simulink library "nonlinearPlnt_cl"  (R2018a)
settings: Solver=VariableStepAuto  StartTime=0.0  StopTime=10.0  RelTol=1e-3
libraries: nonlinearPlnt_ul x1
settings Model: Creator=mcobb  LastModifiedBy=mcobb

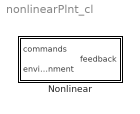
== system nonlinearPlnt_cl ==
  Nonlinear : Subsystem  VariantControl=VSS_NONLINEAR_PLNT

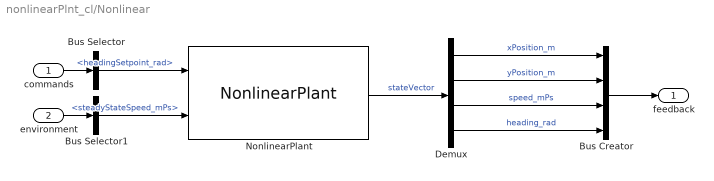
== system nonlinearPlnt_cl/Nonlinear ==
  commands : Inport
  environment : Inport  Port=2
  Bus Creator : BusCreator  Inputs=4
  Bus Selector : BusSelector  OutputSignals=headingSetpoint_rad
  Bus Selector1 : BusSelector  OutputSignals=steadyStateSpeed_mPs
  Demux : Demux
  NonlinearPlant : nonlinearPlnt_ul/NonlinearPlant
  feedback : Outport
  wires:
  Bus Selector1/1 -> NonlinearPlant/2  "<steadyStateSpeed_mPs>"
  Bus Selector/1 -> NonlinearPlant/1  "<headingSetpoint_rad>"
  commands/1 -> Bus Selector/1
  environment/1 -> Bus Selector1/1
  Bus Creator/1 -> feedback/1
  NonlinearPlant/1 -> Demux/1  "stateVector"
  Demux/1 -> Bus Creator/1  "xPosition_m"
  Demux/2 -> Bus Creator/2  "yPosition_m"
  Demux/3 -> Bus Creator/3  "speed_mPs"
  Demux/4 -> Bus Creator/4  "heading_rad"
